simulink model "LMPC"  (R2023b)
settings: Solver=VariableStepAuto  StartTime=0.0  StopTime=inf  RelTol=1e-3
undefined symbols (not defined in the file or in its folder): CoordinateFrame, TypeMask, Velocity, YawRate
libraries: robotlib x3, mpclib x1, aerolibanimutils x1
settings Model: Creator=oem  LastModifiedBy=farhan

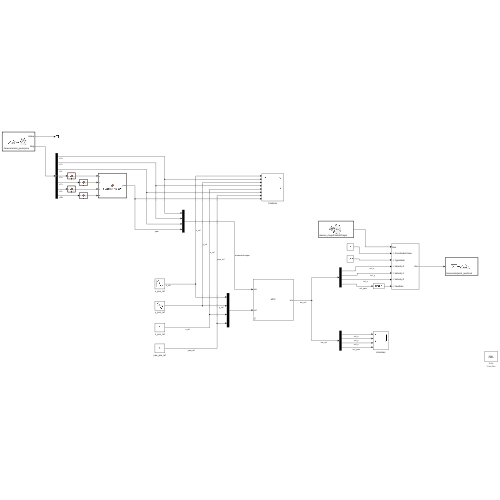
[thumbnail: Simulink's stored preview of the top-level diagram]
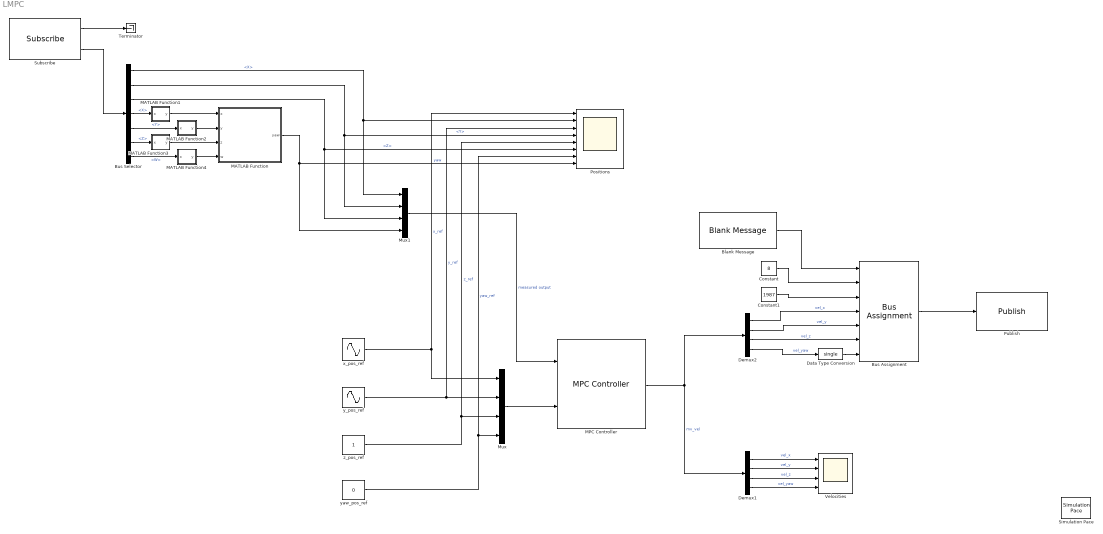
== system LMPC ==
  Blank Message : robotlib/Blank Message  messageClass=Message  entityType=mavros_msgs/PositionTarget  messageType=mavros_msgs/PositionTarget  SampleTime=inf  legacyBusStruct=off
  Bus Assignment : BusAssignment  AssignedSignals=CoordinateFrame,TypeMask,Velocity.X,Velocity.Y,Velocity.Z,YawRate
  Bus Selector : BusSelector  OutputSignals=Pose.Position.X,Pose.Position.Y,Pose.Position.Z,Pose.Orientation.X,Pose.Orientation.Y,Pose.Orientation.Z,Pose.Orientation.W
  Constant : Constant  Value=8  OutDataTypeStr=uint8
  Constant1 : Constant  Value=1987  OutDataTypeStr=uint16
  Data Type Conversion : DataTypeConversion  OutDataTypeStr=single  SaturateOnIntegerOverflow=off  RndMeth=Floor
  Demux1 : Demux
  Demux2 : Demux
  MATLAB Function : MATLAB Function  TreatAsAtomicUnit=on
  MATLAB Function1 : MATLAB Function  TreatAsAtomicUnit=on
  MATLAB Function2 : MATLAB Function  TreatAsAtomicUnit=on
  MATLAB Function3 : MATLAB Function  TreatAsAtomicUnit=on
  MATLAB Function4 : MATLAB Function  TreatAsAtomicUnit=on
  MPC Controller : mpclib/MPC Controller  SCDEnableBlockLinearizationSpecification=on  mpcobj=mpc1  is_multiple=0  enable_value=0  return_u0=off  updateMPCinCallerWorkspace=on  md_inport=off  mv_inport=off  uref_inport=off  return_cost=off  return_mvseq=off  return_qpstatus=off  return_xseq=off  return_state=off  return_ovseq=off  state_inport=off  umin_inport=off  umax_inport=off  ymin_inport=off  ymax_inport=off  cc_inport=off  ywt_inport=off  uwt_inport=off  duwt_inport=off  rhoeps_inport=off  pm_inport=off  MaximumP=10  HorizonChoice=FixedHorizon  n_ts=0.1  n_p=6  n_mv=4  n_md=0  n_ud=0  n_mo=4  n_uo=0  BlockDataType=double  SampleTimeInherited=off  switch_inport=off
  Mux : Mux
  Mux1 : Mux
  Positions : Scope  NumInputPorts=8
  Publish : robotlib/Publish  topicSource=Select from ROS network  topic=/mavros/setpoint_raw/local  messageType=mavros_msgs/PositionTarget  legacyBusStruct=off  messageQueueLength=1
  Simulation Pace : aerolibanimutils/Simulation Pace  SimulationPace=1  SleepMode=Auto  OutputPaceError=off  SampleTime=1/30
  Subscribe : robotlib/Subscribe  topicSource=Select from ROS network  topic=/mavros/vision_pose/pose  messageType=geometry_msgs/PoseStamped  SampleTime=-1  legacyBusStruct=off  messageQueueLength=1
  Terminator : Terminator
  Velocities : Scope  NumInputPorts=4
  x_pos_ref : Sin  Bias=2.33  Frequency=0.4  SampleTime=0
  y_pos_ref : Sin  Bias=2.55  Frequency=0.4  Phase=pi/2  SampleTime=0
  yaw_pos_ref : Constant  Value=0
  z_pos_ref : Constant
  wires:
  MPC Controller/1 -> Demux2/1, Demux1/1  "mv_vel"
  Mux/1 -> MPC Controller/2
  x_pos_ref/1 -> Mux/1, Positions/1  "x_ref"
  y_pos_ref/1 -> Positions/3, Mux/2  "y_ref"
  z_pos_ref/1 -> Positions/5, Mux/3  "z_ref"
  yaw_pos_ref/1 -> Positions/7, Mux/4  "yaw_ref"
  Demux1/1 -> Velocities/1  "vel_x"
  Demux1/2 -> Velocities/2  "vel_y"
  Demux1/3 -> Velocities/3  "vel_z"
  Demux1/4 -> Velocities/4  "vel_yaw"
  Blank Message/1 -> Bus Assignment/1
  Constant/1 -> Bus Assignment/2
  Constant1/1 -> Bus Assignment/3
  Demux2/1 -> Bus Assignment/4  "vel_x"
  Demux2/2 -> Bus Assignment/5  "vel_y"
  Demux2/3 -> Bus Assignment/6  "vel_z"
  Demux2/4 -> Data Type Conversion/1  "vel_yaw"
  Data Type Conversion/1 -> Bus Assignment/7
  Bus Assignment/1 -> Publish/1
  Subscribe/1 -> Terminator/1
  Subscribe/2 -> Bus Selector/1
  Mux1/1 -> MPC Controller/1  "measured output"
  Bus Selector/1 -> Mux1/1, Positions/2  "<X>"
  Bus Selector/2 -> Mux1/2, Positions/4  "<Y>"
  Bus Selector/3 -> Mux1/3, Positions/6  "<Z>"
  Bus Selector/4 -> MATLAB Function1/1(x)  "<X>"
  Bus Selector/5 -> MATLAB Function2/1(x)  "<Y>"
  Bus Selector/6 -> MATLAB Function3/1(x)  "<Z>"
  Bus Selector/7 -> MATLAB Function4/1(x)  "<W>"
  MATLAB Function/1(yaw) -> Mux1/4, Positions/8  "yaw"
  MATLAB Function1/1(y) -> MATLAB Function/1(x)
  MATLAB Function2/1(y) -> MATLAB Function/2(y)
  MATLAB Function3/1(y) -> MATLAB Function/3(z)
  MATLAB Function4/1(y) -> MATLAB Function/4(w)

== matlab function LMPC/MATLAB Function1 ==
  data: x input; y output
function y = f(x)
    % Round off the input number to two decimal places
    y = round(x * 100) / 100;
end

== matlab function LMPC/MATLAB Function ==
  data: x input; yaw output; y input; z input; w input
function yaw = quaternionToYaw(x, y, z, w)
    % Convert quaternion to yaw angle
    q = quaternion(w, x, y, z); % Create quaternion object
    % Convert quaternion to rotation matrix
    rotMat = quat2rotm(q);
    % Extract yaw angle from rotation matrix
    yaw = atan2(rotMat(2,1), rotMat(1,1));
    % Convert yaw angle to degrees
    yaw = rad2deg(yaw);
end

== matlab function LMPC/MATLAB Function2 ==
  data: x input; y output
function y = f(x)
    % Round off the input number to two decimal places
    y = round(x * 100) / 100;
end

== matlab function LMPC/MATLAB Function3 ==
  data: x input; y output
function y = f(x)
    % Round off the input number to two decimal places
    y = round(x * 100) / 100;
end

== matlab function LMPC/MATLAB Function4 ==
  data: x input; y output
function y = f(x)
    % Round off the input number to two decimal places
    y = round(x * 100) / 100;
end
